simulink model "midterm"  (R2013a)
settings: Solver=FixedStepDiscrete  StartTime=0.0  StopTime=10*ms  FixedStep=Ts  RelTol=1e-3
InitFcn:
  | ms=1e-3;
  | KHz=1e3;
  | F1=22*KHz;
  | F2=45*KHz;
  | Fs=200*KHz;
  | Ts=1/Fs;
  | N=1024;
undefined symbols (not defined in the file or in its folder): get
libraries: dspxfrm3 x1, dspsnks4 x1, dspsigops x1
settings Model: Creator=Lee  LastModifiedBy=cory

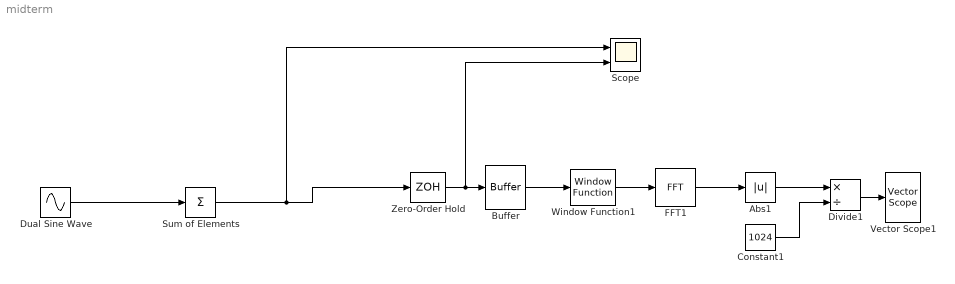
== system midterm ==
  Abs1 : Abs
  Buffer : Buffer  N=1024  TreatMby1Signals=One channel
  Constant1 : Constant  Value=1024
  Divide1 : Product  Inputs=*/
  Dual Sine Wave : Sin  Amplitude=[0.5, 1]  Bias=[0, 0]  Frequency=2*pi*[22, 45]*1e3  Phase=[pi/2, 0]  SampleTime=0
  FFT1 : dspxfrm3/FFT  CompMethod=Table lookup  TableOpt=NEW  TableOptActive=Speed  BitRevOrder=off  InheritFFTLength=on  FFTLength=64  RowConvenienceOn=on  FFTImplementation=Auto  SkipNorm=off  firstCoeffDataTypeStr=Inherit: Same word length as input  firstCoeffLastDataTypeStr=Inherit: Same word length as input  outputMin=[]  outputMax=[]  roundingMode=Floor  overflowMode=off
  Scope : Scope  NumInputPorts=2
      settings: TimeRange=0.0001  YMin=-0.90625~-5  YMax=1.15625~5
  Sum of Elements : Sum  Inputs=+
  Vector Scope1 : dspsnks4/Vector Scope  ScopeProperties=on  Domain=Frequency  HorizSpan=1  DisplayProperties=off  AxisGrid=on  Memory=off  FrameNumber=on  AxisLegend=off  AxisZoom=off  OpenScopeAtSimStart=on  OpenScopeImmediately=off  FigPos=get(0,'defaultfigureposition')  AxisProperties=off  XUnits=Hertz  XRange=[0...Fs/2]  InheritXIncr=on  XIncr=1  XLabel=Time  XLimit=Auto  XMin=0  XMax=1  XStart=0  YUnits=dB  YLabel=Amplitude  LineProperties=off  XAxisParamsVer=6.9
      settings: YMin=-30  YMax=1
  Window Function1 : dspsigops/Window Function  winmode=Apply window to input  wintype=Bartlett  sampmode=Continuous  samptime=1  N=64  Rs=50  beta=10  winsamp=Symmetric  UserWindow=hamming  OptParams=off  UserParams={'symmetric'}  RowConvenienceOn=on  dataType=double  isSigned=on  wordLen=16  udDataType=sfix(16)  fracBitsMode=Best precision  numFracBits=15  roundingMode=Floor  overflowMode=off  numSidelobes=4  sidelobeLevel=-30
  Zero-Order Hold : ZeroOrderHold  SampleTime=Ts
  wires:
  Zero-Order Hold/1 -> Scope/2, Buffer/1
  FFT1/1 -> Abs1/1
  Constant1/1 -> Divide1/2
  Abs1/1 -> Divide1/1
  Divide1/1 -> Vector Scope1/1
  Buffer/1 -> Window Function1/1
  Window Function1/1 -> FFT1/1
  Dual Sine Wave/1 -> Sum of Elements/1
  Sum of Elements/1 -> Scope/1, Zero-Order Hold/1
